simulink model "OpenLoop_SIM"  (R2018b)
settings: Solver=FixedStepDiscrete  StartTime=start_time  StopTime=IMU.timestamp.Time(end)  FixedStep=0.002  RelTol=1e-3
settings Model: SimulationMode=accelerator  Creator=M18001  LastModifiedBy=zouji
settings OptimizationCC: DefaultUnderspecifiedDataType=single  EfficientMapNaN2IntZero=off
settings DebuggingCC: ParameterOverflowMsg=none  UnconnectedInputMsg=none  UnconnectedOutputMsg=none  UnconnectedLineMsg=none
settings HardwareCC: TargetBitPerPointer=64  TargetBitPerSizeT=64  TargetBitPerPtrDiffT=64  TargetLongLongMode=on  TargetIntDivRoundTo=Zero  TargetEndianess=LittleEndian  TargetWordSize=64  TargetHWDeviceType=MATLAB Host  ProdEqTarget=off
settings ModelReferenceCC: ModelReferenceNumInstancesAllowed=Single
settings CodeAppCC: MaxIdLength=128
settings GRTTargetCC: TargetLangStandard=C89/C90 (ANSI)  CombineOutputUpdateFcns=off  GRTInterface=on

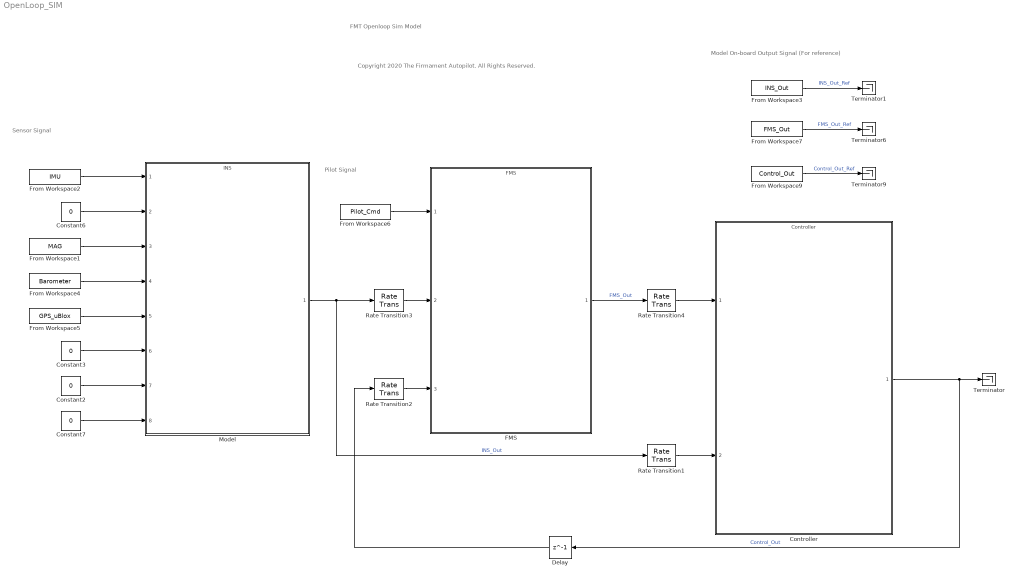
== system OpenLoop_SIM ==
  note: Pilot Signal
  note: Sensor Signal
  note: Model On-board Output Signal (For reference)
  note: FMT Openloop Sim Model
  note: Copyright 2020 The Firmament Autopilot. All Rights Reserved.
  Constant2 : Constant  Value=0  OutDataTypeStr=Bus: Optical_Flow_Bus
  Constant3 : Constant  Value=0  OutDataTypeStr=Bus: Sonar_Bus
  Constant6 : Constant  Value=0  OutDataTypeStr=Bus: IMU_Bus
  Constant7 : Constant  Value=0  OutDataTypeStr=uint8
  Controller : ModelReference  ModelNameDialog=Controller.slx  ModelReferenceVersion=1.582
  Delay : Delay  DelayLength=1
  FMS : ModelReference  ModelNameDialog=FMS.slx  ModelReferenceVersion=1.622
  From Workspace1 : FromWorkspace  VariableName=MAG  OutDataTypeStr=Bus: MAG_Bus  Interpolate=off  OutputAfterFinalValue=Holding final value
  From Workspace2 : FromWorkspace  VariableName=IMU  OutDataTypeStr=Bus: IMU_Bus  Interpolate=off  OutputAfterFinalValue=Holding final value
  From Workspace3 : FromWorkspace  VariableName=INS_Out  OutDataTypeStr=Bus: INS_Out_Bus  Interpolate=off  OutputAfterFinalValue=Holding final value
  From Workspace4 : FromWorkspace  VariableName=Barometer  OutDataTypeStr=Bus: Barometer_Bus  Interpolate=off  OutputAfterFinalValue=Holding final value
  From Workspace5 : FromWorkspace  VariableName=GPS_uBlox  OutDataTypeStr=Bus: GPS_uBlox_Bus  Interpolate=off  OutputAfterFinalValue=Holding final value
  From Workspace6 : FromWorkspace  VariableName=Pilot_Cmd  OutDataTypeStr=Bus: Pilot_Cmd_Bus  Interpolate=off  OutputAfterFinalValue=Holding final value
  From Workspace7 : FromWorkspace  VariableName=FMS_Out  OutDataTypeStr=Bus: FMS_Out_Bus  Interpolate=off  OutputAfterFinalValue=Holding final value
  From Workspace9 : FromWorkspace  VariableName=Control_Out  OutDataTypeStr=Bus: Control_Out_Bus  Interpolate=off  OutputAfterFinalValue=Holding final value
  Model : ModelReference  ModelNameDialog=INS.slx  ModelReferenceVersion=1.2562
  Rate Transition1 : RateTransition  OutPortSampleTime=CONTROL_CONST.dt
  Rate Transition2 : RateTransition  OutPortSampleTime=FMS_CONST.dt
  Rate Transition3 : RateTransition  OutPortSampleTime=FMS_CONST.dt
  Rate Transition4 : RateTransition  OutPortSampleTime=CONTROL_CONST.dt
  Terminator{,1,6,9} (4 alike) : Terminator
  wires:
  From Workspace2/1 -> Model/1
  Constant6/1 -> Model/2
  From Workspace1/1 -> Model/3
  From Workspace5/1 -> Model/5
  Constant2/1 -> Model/7
  Constant3/1 -> Model/6
  Constant7/1 -> Model/8
  From Workspace3/1 -> Terminator1/1  "INS_Out_Ref"
  From Workspace4/1 -> Model/4
  Rate Transition3/1 -> FMS/2
  Rate Transition1/1 -> Controller/2
  Model/1 -> Rate Transition3/1, Rate Transition1/1  "INS_Out"
  FMS/1 -> Rate Transition4/1  "FMS_Out"
  From Workspace6/1 -> FMS/1
  Controller/1 -> Delay/1, Terminator/1  "Control_Out"
  From Workspace7/1 -> Terminator6/1  "FMS_Out_Ref"
  From Workspace9/1 -> Terminator9/1  "Control_Out_Ref"
  Rate Transition2/1 -> FMS/3
  Delay/1 -> Rate Transition2/1
  Rate Transition4/1 -> Controller/1
